simulink model "Sum_Lab"  (R2024b)
settings: Solver=VariableStepAuto  StartTime=0.0  StopTime=10.0  RelTol=1e-3
settings Model: Creator=Ahmad  LastModifiedBy=Ahmad

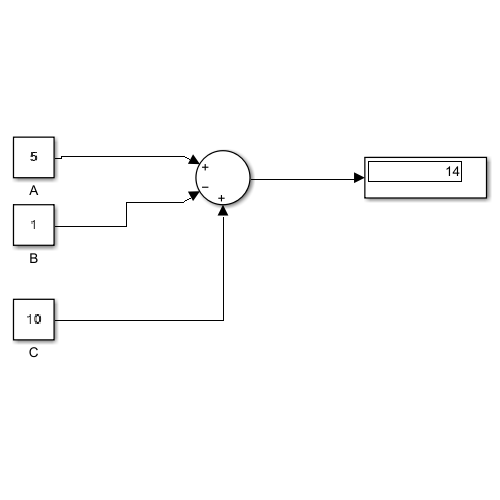
[thumbnail: Simulink's stored preview of the top-level diagram]
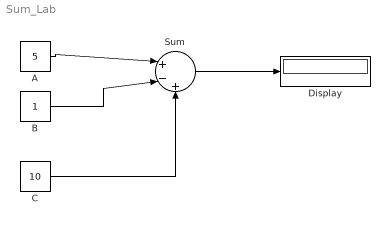
== system Sum_Lab ==
  A : Constant  Value=5
  B : Constant
  C : Constant  Value=10
  Display : Display
  Sum : Sum  Inputs=|+-+
  wires:
  A/1 -> Sum/1
  B/1 -> Sum/2
  Sum/1 -> Display/1
  C/1 -> Sum/3
